simulink model "MATLAB_pendulum_model"  (R2014a)
settings: Solver=ode45  StartTime=0.0  StopTime=10.0  RelTol=1e-3
values from neighbouring files (symbols this model uses):
  b = 0.1    [MATLAB_pendulum_init.m]
  g = 9.81    [MATLAB_pendulum_init.m]
  I = 0.006    [MATLAB_pendulum_init.m]
  l = 0.3    [MATLAB_pendulum_init.m]
  M = 0.5    [MATLAB_pendulum_init.m]
  m = 0.2    [MATLAB_pendulum_init.m]
settings Model: Creator=Ash  LastModifiedBy=Ash
settings SolverCC: AlgebraicLoopSolver=LineSearch

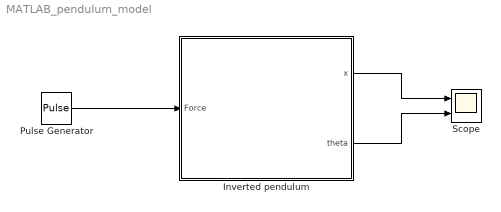
== system MATLAB_pendulum_model ==
  Inverted pendulum : Subsystem
  Pulse Generator : DiscretePulseGenerator  PulseType=Time based  Amplitude=1000  Period=10  PulseWidth=0.01
  Scope : Scope  NumInputPorts=2
      settings: YMin=-5~-5  YMax=5~5
  wires:
  Pulse Generator/1 -> Inverted pendulum/1(Force)
  Inverted pendulum/1(x) -> Scope/1
  Inverted pendulum/2(theta) -> Scope/2

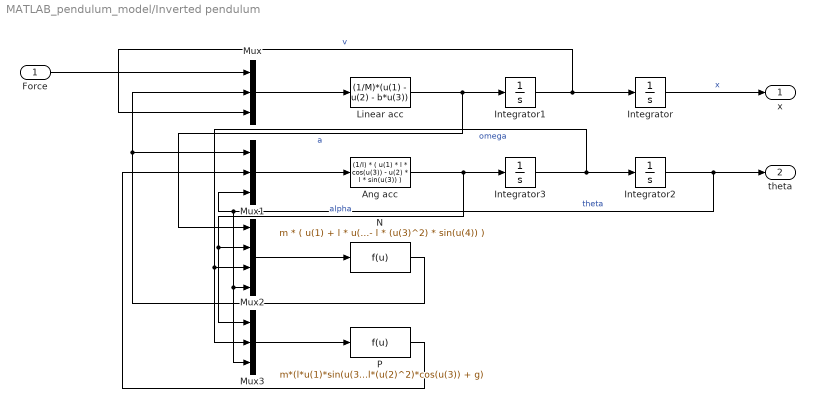
== system MATLAB_pendulum_model/Inverted pendulum ==
  Force : Inport
  "Ang acc " : Fcn  Expr=(1/I) * ( u(1) * l * cos(u(3)) - u(2) * l * sin(u(3)) )
  Integrator : Integrator  ContinuousStateAttributes='x'
  Integrator1 : Integrator  ContinuousStateAttributes='v'
  Integrator2 : Integrator  InitialCondition=pi  ContinuousStateAttributes='theta'
  Integrator3 : Integrator  ContinuousStateAttributes='omega'
  Linear acc : Fcn  Expr=(1/M)*(u(1) - u(2) - b*u(3))
  Mux : Mux  Inputs=3
  Mux1 : Mux  Inputs=3
  Mux2 : Mux
  Mux3 : Mux  Inputs=3
  N : Fcn  Expr=m * ( u(1) + l * u(2) * cos(u(4)) - l * (u(3)^2) * sin(u(4)) )
  P : Fcn  Expr=m*(l*u(1)*sin(u(3)) + l*(u(2)^2)*cos(u(3)) + g)
  x : Outport
  theta : Outport  Port=2
  wires:
  Mux1/1 -> "Ang acc "/1
  Linear acc/1 -> Mux2/1, Integrator1/1  "a"
  Force/1 -> Mux/1
  N/1 -> Mux1/1, Mux/2
  Integrator3/1 -> Mux3/2, Mux2/3, Integrator2/1  "omega"
  Integrator2/1 -> theta/1, Mux3/3, Mux2/4, Mux1/3  "theta"
  Mux2/1 -> N/1
  "Ang acc "/1 -> Mux3/1, Mux2/2, Integrator3/1  "alpha"
  Integrator/1 -> x/1  "x"
  Mux/1 -> Linear acc/1
  Mux3/1 -> P/1
  Integrator1/1 -> Mux/3, Integrator/1  "v"
  P/1 -> Mux1/2
